simulink model "Automatic_Braking_System"  (R2025a)
settings: Solver=VariableStepAuto  StartTime=0.0  StopTime=20  RelTol=1e-3
settings Model: Creator=Rudransh  LastModifiedBy=Rudransh

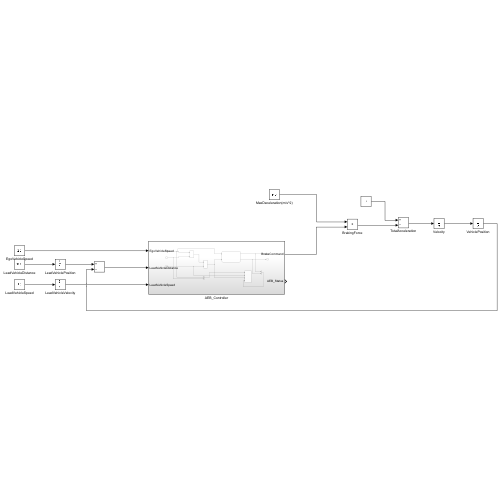
[thumbnail: Simulink's stored preview of the top-level diagram]
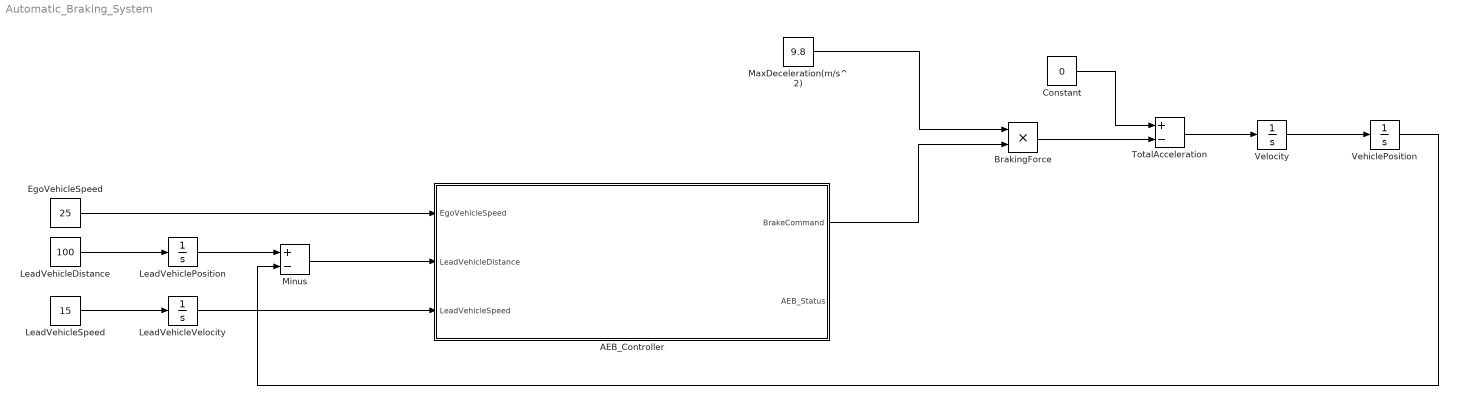
== system Automatic_Braking_System ==
  AEB_Controller : Subsystem
  BrakingForce : Product
  Constant : Constant  Value=0
  EgoVehicleSpeed : Constant  Value=25
  LeadVehicleDistance : Constant  Value=100
  LeadVehiclePosition : Integrator  InitialCondition=100
  LeadVehicleSpeed : Constant  Value=15
  LeadVehicleVelocity : Integrator  InitialCondition=15
  MaxDeceleration(m/s^2) : Constant  Value=9.8
  Minus : Sum  Inputs=+-
  TotalAcceleration : Sum  Inputs=+-
  VehiclePosition : Integrator
  Velocity : Integrator  InitialCondition=25
  wires:
  AEB_Controller/1(BrakeCommand) -> BrakingForce/2
  MaxDeceleration(m/s^2)/1 -> BrakingForce/1
  BrakingForce/1 -> TotalAcceleration/2
  Constant/1 -> TotalAcceleration/1
  TotalAcceleration/1 -> Velocity/1
  Velocity/1 -> VehiclePosition/1
  LeadVehicleSpeed/1 -> LeadVehicleVelocity/1
  LeadVehicleVelocity/1 -> AEB_Controller/3(LeadVehicleSpeed)
  LeadVehicleDistance/1 -> LeadVehiclePosition/1
  LeadVehiclePosition/1 -> Minus/1
  Minus/1 -> AEB_Controller/2(LeadVehicleDistance)
  VehiclePosition/1 -> Minus/2
  EgoVehicleSpeed/1 -> AEB_Controller/1(EgoVehicleSpeed)

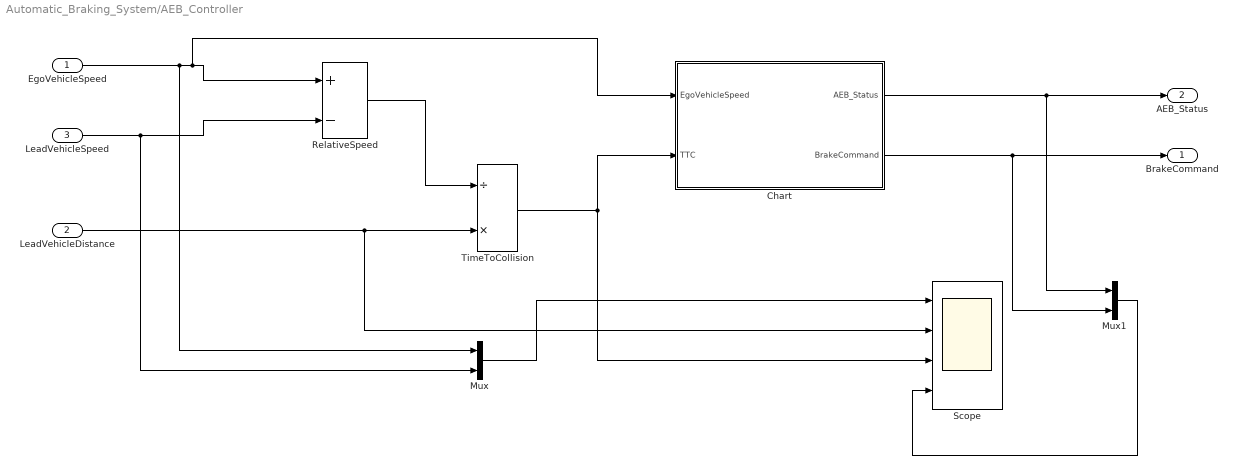
== system Automatic_Braking_System/AEB_Controller ==
  EgoVehicleSpeed : Inport
  LeadVehicleDistance : Inport  Port=2
  LeadVehicleSpeed : Inport  Port=3
  Chart : Stateflow chart  TreatAsAtomicUnit=on
  Mux : Mux  Inputs=2
  Mux1 : Mux  Inputs=2
  RelativeSpeed : Sum  Inputs=+-
  Scope : Scope  NumInputPorts=4
      settings: ActiveDisplayString=4  ActiveDisplayYMinimum=-1  ActiveDisplayYMaximum=3
  TimeToCollision : Product  Inputs=/*
  BrakeCommand : Outport
  AEB_Status : Outport  Port=2
  wires:
  EgoVehicleSpeed/1 -> Mux/1, Chart/1(EgoVehicleSpeed), RelativeSpeed/1
  LeadVehicleSpeed/1 -> Mux/2, RelativeSpeed/2
  LeadVehicleDistance/1 -> Scope/2, TimeToCollision/2
  RelativeSpeed/1 -> TimeToCollision/1
  TimeToCollision/1 -> Scope/3, Chart/2(TTC)
  Chart/1(AEB_Status) -> Mux1/1, AEB_Status/1
  Chart/2(BrakeCommand) -> Mux1/2, BrakeCommand/1
  Mux/1 -> Scope/1
  Mux1/1 -> Scope/4

== stateflow chart Automatic_Braking_System/AEB_Controller/Chart ==
  state Safe
    entry: BrakeCommand = 0;
    AEB_Status = 0;
  state Warning
    entry: BrakeCommand = 0;
    AEB_Status = 1;
  state Braking
    entry: BrakeCommand = 1;
    AEB_Status = 2;
  (default) -> Safe
  Braking -> Safe : [EgoVehicleSpeed < 0.1]
  Safe -> Warning : [TTC < 2.5]
  Warning -> Safe [order 2] : [TTC >= 2.5]
  Warning -> Braking [order 1] : [TTC < 1.2]
  data: EgoVehicleSpeed input; AEB_Status output; BrakeCommand output; TTC input
